simulink model "untitled"  (Simulink 7.9)
settings: Solver=VariableStepDiscrete  StartTime=0.0  StopTime=1000.0  RelTol=1e-3
undefined symbols (not defined in the file): des, gcbh
settings Model: Creator=tsprock3  LastModifiedBy=tsprock3

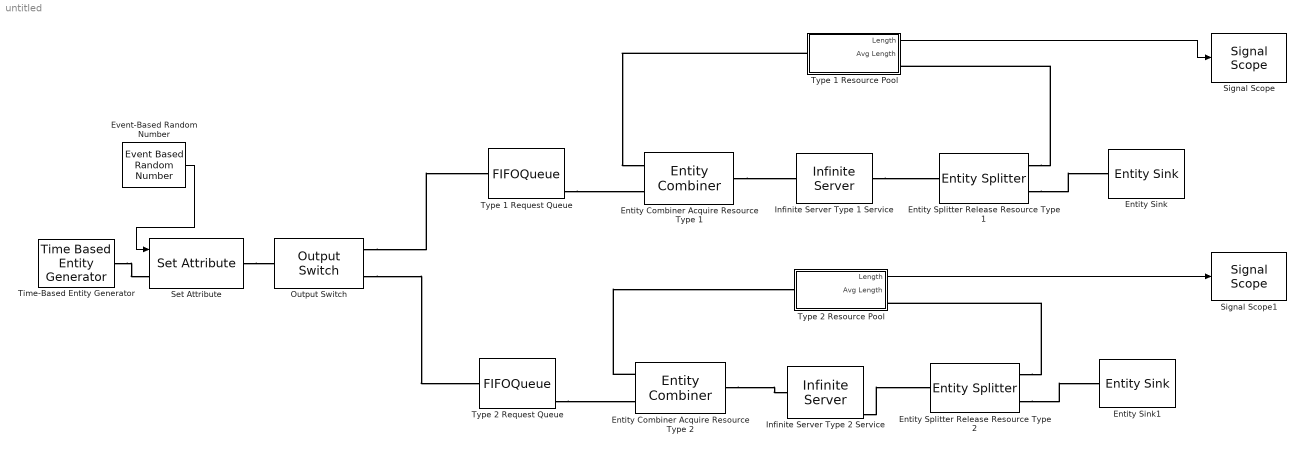
== system untitled ==
  Entity Combiner Acquire Resource Type 1 : EntityCombiner  NumberInputPorts=2
  Entity Combiner Acquire Resource Type 2 : EntityCombiner  NumberInputPorts=2
  Entity Sink : EntitySink
  Entity Sink1 : EntitySink
  Entity Splitter Release Resource Type 1 : EntitySplitter  NumberOutputPorts=2
  Entity Splitter Release Resource Type 2 : EntitySplitter  NumberOutputPorts=2
  Event-Based Random Number : EventBasedRandomNumber  Distribution=Arbitrary discrete  pOneBern=0.4  minUnid=1  maxUnid=2  valueVecDisc=[1 2]  probVecDisc=[0.4 0.6]
  Infinite Server Type 1 Service : InfiniteServer  ServiceTime=0.05
  Infinite Server Type 2 Service : InfiniteServer  ServiceTime=0.5  StatNumberDeparted=on  StatNumberInBlock=on  StatPendingEntity=on  StatNumberPending=on  StatAverageWait=on  StatNumberTimedout=on
      settings: OutputPortMap=o0,o1,o2,o3,o4,o5
  Output Switch : OutputSwitch  NumberOutputPorts=2  SwitchingCriterion=From attribute  AttributeName=RequestType
  Set Attribute : SetAttribute  AttributeName=RequestType  AttributeFrom=Signal port  EvaluatedAttributeValue={[]}
  Signal Scope : SignalScope  LoadFcn=des.scope.CallbackSupport('seLoadFcn',gcbh)  StartFcn=des.scope.CallbackSupport('seStartFcn',gcbh)  StopFcn=des.scope.CallbackSupport('seStopFcn',gcbh)
      settings: CopyFcn=des.scope.CallbackSupport('seCopyFcn',gcbh)  DeleteFcn=des.scope.CallbackSupport('seDeleteFcn',gcbh)  PreSaveFcn=des.scope.CallbackSupport('sePreSaveFcn',gcbh)  NameChangeFcn=des.scope.CallbackSupport('seNameChangeFcn',gcbh)  OpenFcn=des.scope.CallbackSupport('seOpenFcn',gcbh)
  Signal Scope1 : SignalScope  LoadFcn=des.scope.CallbackSupport('seLoadFcn',gcbh)  StartFcn=des.scope.CallbackSupport('seStartFcn',gcbh)  StopFcn=des.scope.CallbackSupport('seStopFcn',gcbh)
      settings: CopyFcn=des.scope.CallbackSupport('seCopyFcn',gcbh)  DeleteFcn=des.scope.CallbackSupport('seDeleteFcn',gcbh)  PreSaveFcn=des.scope.CallbackSupport('sePreSaveFcn',gcbh)  NameChangeFcn=des.scope.CallbackSupport('seNameChangeFcn',gcbh)  OpenFcn=des.scope.CallbackSupport('seOpenFcn',gcbh)
  Time-Based Entity Generator : TimeBasedEntityGenerator  Distribution=Uniform  Maximum=0.5
  Type 1 Request Queue : FIFOQueue  StatNumberInBlock=on  StatAverageWait=on
      settings: OutputPortMap=o1,o2
  Type 1 Resource Pool : Subsystem
  Type 2 Request Queue : FIFOQueue  StatNumberInBlock=on  StatAverageWait=on
      settings: OutputPortMap=o1,o2
  Type 2 Resource Pool : Subsystem
  wires:
  Event-Based Random Number/1 -> Set Attribute/1
  Type 1 Resource Pool/1(Length) -> Signal Scope/1
  Type 2 Resource Pool/1(Length) -> Signal Scope1/1
  connections:
  Time-Based Entity Generator/RConn1 -- Set Attribute/LConn1
  Set Attribute/RConn1 -- Output Switch/LConn1
  Entity Splitter Release Resource Type 1/RConn2 -- Entity Sink/LConn1
  Entity Splitter Release Resource Type 1/RConn1 -- Type 1 Resource Pool/RConn1
  Infinite Server Type 1 Service/RConn1 -- Entity Splitter Release Resource Type 1/LConn1
  Entity Combiner Acquire Resource Type 1/RConn1 -- Infinite Server Type 1 Service/LConn1
  Type 1 Request Queue/RConn1 -- Entity Combiner Acquire Resource Type 1/LConn2
  Infinite Server Type 2 Service/RConn1 -- Entity Splitter Release Resource Type 2/LConn1
  Entity Combiner Acquire Resource Type 2/RConn1 -- Infinite Server Type 2 Service/LConn1
  Entity Splitter Release Resource Type 2/RConn1 -- Type 2 Resource Pool/RConn1
  Type 2 Request Queue/RConn1 -- Entity Combiner Acquire Resource Type 2/LConn2
  Entity Combiner Acquire Resource Type 2/LConn1 -- Type 2 Resource Pool/LConn1
  Entity Splitter Release Resource Type 2/RConn2 -- Entity Sink1/LConn1
  Output Switch/RConn1 -- Type 1 Request Queue/LConn1
  Output Switch/RConn2 -- Type 2 Request Queue/LConn1
  Type 1 Resource Pool/LConn1 -- Entity Combiner Acquire Resource Type 1/LConn1

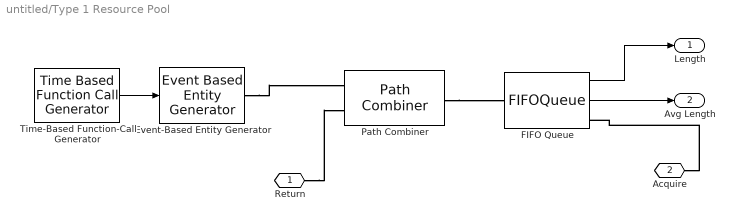
== system untitled/Type 1 Resource Pool ==
  Event-Based Entity Generator : EventBasedEntityGenerator  GenerateEntitiesUpon=Function call from port fcn
  FIFO Queue : FIFOQueue  Capacity=5  StatNumberInBlock=on  StatAverageQueueLength=on
      settings: OutputPortMap=o1,o3
  Path Combiner : PathCombiner  NumberInputPorts=2
  Time-Based Function-Call Generator : TimeBasedFunctionCallGenerator  EventGenerationMode=Only at simulation start  NumberOfEventsPerPeriod=4
  Return : PMIOPort  Port=1  Side=Right
  Acquire : PMIOPort  Port=2  Side=Left
  Length : Outport
  Avg Length : Outport  Port=2
  wires:
  Time-Based Function-Call Generator/1 -> Event-Based Entity Generator/1
  FIFO Queue/2 -> Avg Length/1
  FIFO Queue/1 -> Length/1
  connections:
  Event-Based Entity Generator/RConn1 -- Path Combiner/LConn1
  Path Combiner/RConn1 -- FIFO Queue/LConn1
  Return/RConn1 -- Path Combiner/LConn2
  Acquire/RConn1 -- FIFO Queue/RConn1

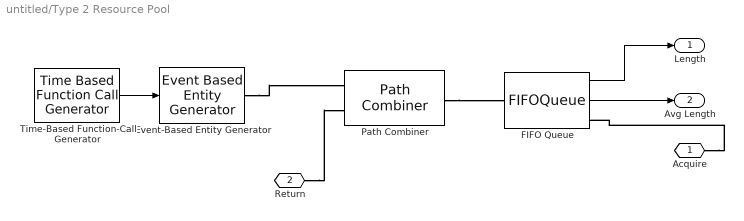
== system untitled/Type 2 Resource Pool ==
  Event-Based Entity Generator : EventBasedEntityGenerator  GenerateEntitiesUpon=Function call from port fcn
  FIFO Queue : FIFOQueue  Capacity=8  StatNumberInBlock=on  StatAverageQueueLength=on
      settings: OutputPortMap=o1,o3
  Path Combiner : PathCombiner  NumberInputPorts=2
  Time-Based Function-Call Generator : TimeBasedFunctionCallGenerator  EventGenerationMode=Only at simulation start  NumberOfEventsPerPeriod=6
  Acquire : PMIOPort  Port=1  Side=Left
  Return : PMIOPort  Port=2  Side=Right
  Length : Outport
  Avg Length : Outport  Port=2
  wires:
  Time-Based Function-Call Generator/1 -> Event-Based Entity Generator/1
  FIFO Queue/2 -> Avg Length/1
  FIFO Queue/1 -> Length/1
  connections:
  Event-Based Entity Generator/RConn1 -- Path Combiner/LConn1
  Path Combiner/RConn1 -- FIFO Queue/LConn1
  Return/RConn1 -- Path Combiner/LConn2
  Acquire/RConn1 -- FIFO Queue/RConn1
